simulink model "FullModel"  (R2025b)
settings: Solver=ode15s  StartTime=0.0  StopTime=0.3  FixedStep=1e-6  MaxStep=1e-5  RelTol=1e-5  EnableMultiTasking=on
InitFcn:
  | Rs=0.42;
  | Ls=0.96e-3;
  | C_phi=92.1952e-3;
  | poles=8;
  | Rload=15;
values from neighbouring files (symbols this model uses):
  DutyCycleBoost = 0.7    [run_specification.m]
  Lm = 27.27e-6    (= 2.727e-05)    [run_specification.m]
  Lsec = Lp    (= 0.00012957)    [run_specification.m]
  Rp = 0.3117    [run_specification.m]
  rpm_speed = 500    [run_specification.m]
libraries: spsSeriesRLCBranchLib x15, spsDiodeLib x11, spsVoltageMeasurementLib x7, spsMosfetLib x6, spsControlledVoltageSourceLib x3, spsCurrentMeasurementLib x2, spsPWMGeneratorDCDCLib x2, spsParallelRLCBranchLib x2, spsGroundLib x1, spspowerguiLib x1
settings Model: Creator=jwjansen  LastModifiedBy=20231741
settings SolverCC: AlgebraicLoopSolver=TrustRegion
settings DataIOCC: LimitDataPoints=on  SaveFormat=Array  ReturnWorkspaceOutputs=off
settings OptimizationCC: ExpressionDepthLimit=2147483647.0  LifeSpan=inf
settings DebuggingCC: UnderspecifiedInitializationDetection=Classic  MergeDetectMultiDrivingBlocksExec=none  SolverPrmCheckMsg=warning  FcnCallInpInsideContextMsg=warning  StateNameClashWarn=warning  SFUnexpectedBacktrackingDiag=warning  SFNoUnconditionalDefaultTransitionDiag=warning  SFExecutionAtInitializationDiag=none  ArithmeticOperatorsInVariantConditions=warning
settings HardwareCC: ProdBitPerPointer=32.0  ProdBitPerSizeT=32.0  ProdBitPerPtrDiffT=32.0  ProdLargestAtomicFloat=None  ProdIntDivRoundTo=Undefined  ProdEndianess=Unspecified  ProdWordSize=32.0  ProdHWDeviceType=32-bit Generic
settings ModelReferenceCC: EnableRefExpFcnMdlSchedulingChecks=on  PropagateSignalLabelsOutOfModel=off
settings SFSimCC: SimUseLocalCustomCode=off  SimParseCustomCode=off  CustomCodeUndefinedFunction=UseInterfaceOnly
settings RTWCC: RTWUseLocalCustomCode=off  GPUComputeCapability=3.5
settings CodeAppCC: StateflowObjectComments=on
settings GRTTargetCC: TargetLangStandard=C89/C90 (ANSI)  CombineOutputUpdateFcns=off  GRTInterface=on
settings ConfigComp: CovMetricSettings=dw  CovSaveCumulativeToWorkspaceVar=on  CovSaveSingleToWorkspaceVar=on  CovExternalEMLEnable=off
settings SimscapeCC: SimscapeNormalizeSystem=off

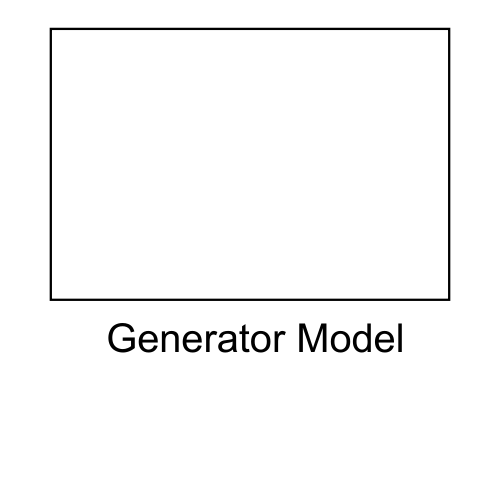
[thumbnail: Simulink's stored preview of the top-level diagram]
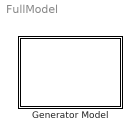
== system FullModel ==
  " Generator Model " : Subsystem

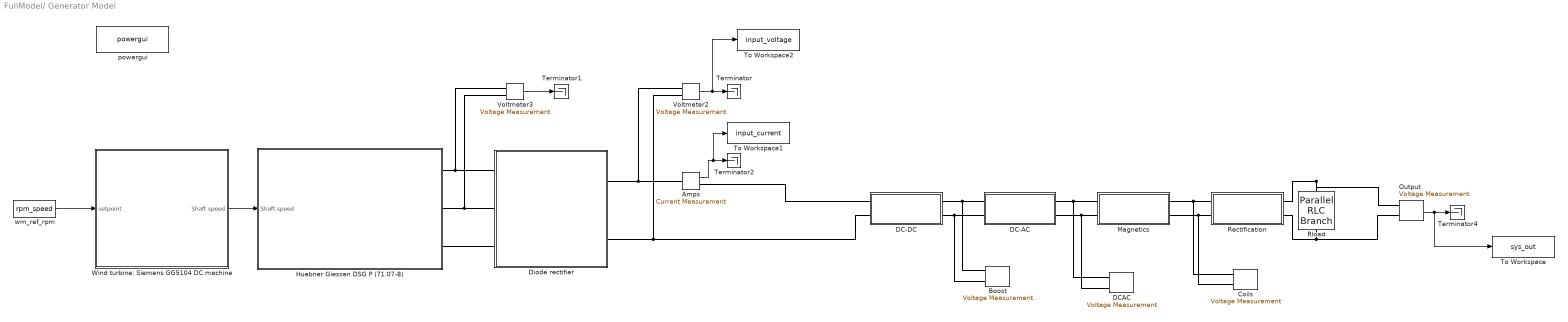
== system FullModel/ Generator Model  ==
  Amps : spsCurrentMeasurementLib/Current Measurement  PhasorSimulation=off  OutputType=Complex  PSBequivalent=0
  Boost : spsVoltageMeasurementLib/Voltage Measurement  PhasorSimulation=off  OutputType=Complex  PSBequivalent=0
  Coils : spsVoltageMeasurementLib/Voltage Measurement  PhasorSimulation=off  OutputType=Complex  PSBequivalent=0
  DC-AC : Subsystem
  DC-DC : Subsystem
  DCAC : spsVoltageMeasurementLib/Voltage Measurement  PhasorSimulation=off  OutputType=Complex  PSBequivalent=0
  Diode rectifier : Subsystem
  "Huebner Giessen DSG P (71.07-8) " : Subsystem
  Magnetics : Subsystem
  Output : spsVoltageMeasurementLib/Voltage Measurement  PhasorSimulation=off  OutputType=Complex  PSBequivalent=0
  Rectification : Subsystem
  Rload : spsParallelRLCBranchLib/Parallel RLC Branch  LConnTagsString=a  RConnTagsString=__new0  BranchType=R  Resistance=9.8  Inductance=0.1e-3  SetiL0=off  InitialCurrent=0  Capacitance=1e-3  Setx0=on  InitialVoltage=14  Measurements=Branch voltage and current
  Terminator{,1..2,4} (4 alike) : Terminator
  To Workspace : ToWorkspace  VariableName=sys_out  SaveFormat=Timeseries  SampleTime=-1
  To Workspace1 : ToWorkspace  VariableName=input_current  SaveFormat=Timeseries  SampleTime=-1
  To Workspace2 : ToWorkspace  VariableName=input_voltage  SaveFormat=Timeseries  SampleTime=-1
  Voltmeter2 : spsVoltageMeasurementLib/Voltage Measurement  PhasorSimulation=off  OutputType=Complex  PSBequivalent=0
  Voltmeter3 : spsVoltageMeasurementLib/Voltage Measurement  PhasorSimulation=off  OutputType=Complex  PSBequivalent=0
  "Wind turbine: Siemens GG5104 DC machine " : Subsystem
  powergui : spspowerguiLib/powergui  Priority=1  SimulationMode=Continuous  SampleTime=1e-6  frequency=60  Iterations=50  frequencyindice=0  Pbase=100e6  ErrMax=1e-4  UnitsV=kV  UnitsW=MW  buscounter=0  FunctionMessages=off  echomessages=off  EnableUseOfTLC=off  CurrentSourceSwitches=off  DisableSnubberDevices=off  DisableRonSwitches=off  DisableVfSwitches=off  DisplayEquations=off  AutomaticDiscreteSolvers=off  SolverType=Tustin  Interpol=off  ExternalGateDelay=off  methode=off  Ts=0  x0status=blocks  SPID=off  SwTol=0  HookPort=off  NonlinearTolerance=1e-4  nMaxIteration=100  ContinueOnMaxIteration=off  RestoreLinks=warning  ResistiveCurrentMeasurement=off  Frange=[0:2:500]  Ylog=off  Xlog=on  ShowGrid=off  save=off  variable=ZData  structure=0  ZoomFFT=off  StartTime=0.0  cycles=1  DisplayStyle=1  fundamental=60  FreqAxis=off  MaxFrequency=1000  frequencyindicesteady=1  RmsSteady=1  display=off
  wm_ref_rpm : Constant  Value=rpm_speed
  wires:
  wm_ref_rpm/1 -> "Wind turbine: Siemens GG5104 DC machine "/1(setpoint)
  "Wind turbine: Siemens GG5104 DC machine "/1(Shaft speed) -> "Huebner Giessen DSG P (71.07-8) "/1(Shaft speed)
  Voltmeter2/1 -> To Workspace2/1, Terminator/1
  Voltmeter3/1 -> Terminator1/1
  Amps/1 -> To Workspace1/1, Terminator2/1
  Output/1 -> To Workspace/1, Terminator4/1
  connections:
  "Huebner Giessen DSG P (71.07-8) "/RConn1 -- Voltmeter3/LConn1 -- Diode rectifier/LConn1
  Diode rectifier/LConn2 -- Voltmeter3/LConn2 -- "Huebner Giessen DSG P (71.07-8) "/RConn2
  Diode rectifier/LConn3 -- "Huebner Giessen DSG P (71.07-8) "/RConn3
  Voltmeter2/LConn1 -- Amps/LConn1 -- Diode rectifier/RConn1
  Voltmeter2/LConn2 -- DC-DC/LConn2 -- Diode rectifier/RConn2
  DC-DC/LConn1 -- Amps/RConn1
  DC-AC/LConn2 -- Boost/LConn2 -- DC-DC/RConn2
  DC-AC/LConn1 -- Boost/LConn1 -- DC-DC/RConn1
  Magnetics/LConn1 -- DCAC/LConn1 -- DC-AC/RConn1
  Magnetics/LConn2 -- DCAC/LConn2 -- DC-AC/RConn2
  Rectification/LConn1 -- Magnetics/RConn1 -- Coils/LConn1
  Rectification/LConn2 -- Magnetics/RConn2 -- Coils/LConn2
  Rload/LConn1 -- Rectification/RConn1 -- Output/LConn1
  Rload/RConn1 -- Rectification/RConn2 -- Output/LConn2

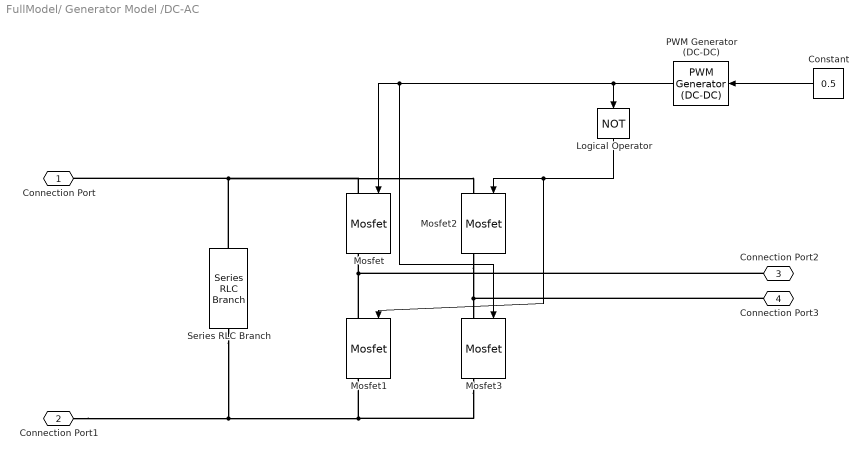
== system FullModel/ Generator Model /DC-AC ==
  Constant : Constant  Value=0.5
  Logical Operator : Logic  Operator=NOT  AllPortsSameDT=off  OutDataTypeStr=boolean
  Mosfet{,1..3} (4 alike) : spsMosfetLib/Mosfet  Ron=90e-3  Lon=0  Rd=0.01  Vfd=0.9  IC=0  Rs=1e5  Cs=inf  Measurements=on
  PWM Generator (DC-DC) : spsPWMGeneratorDCDCLib/PWM Generator (DC-DC)  Fsw=Finv  Ts=0
  Series RLC Branch : spsSeriesRLCBranchLib/Series RLC Branch  LConnTagsString=__new0  RConnTagsString=__new0  BranchType=C  Resistance=1  Inductance=1e-3  SetiL0=off  InitialCurrent=0  Capacitance=470e-6  Setx0=off  InitialVoltage=0  Measurements=None
  Connection Port : PMIOPort  Side=Left
  Connection Port1 : PMIOPort  Port=2  Side=Left
  Connection Port2 : PMIOPort  Port=3  Side=Right
  Connection Port3 : PMIOPort  Port=4  Side=Right
  wires:
  PWM Generator (DC-DC)/1 -> Logical Operator/1, Mosfet3/1, Mosfet/1
  Logical Operator/1 -> Mosfet1/1, Mosfet2/1
  Constant/1 -> PWM Generator (DC-DC)/1
  connections:
  Connection Port1/RConn1 -- Series RLC Branch/RConn1 -- Mosfet3/RConn1 -- Mosfet1/RConn1
  Mosfet2/LConn1 -- Mosfet/LConn1 -- Series RLC Branch/LConn1 -- Connection Port/RConn1
  Connection Port2/RConn1 -- Mosfet/RConn1 -- Mosfet1/LConn1
  Connection Port3/RConn1 -- Mosfet2/RConn1 -- Mosfet3/LConn1

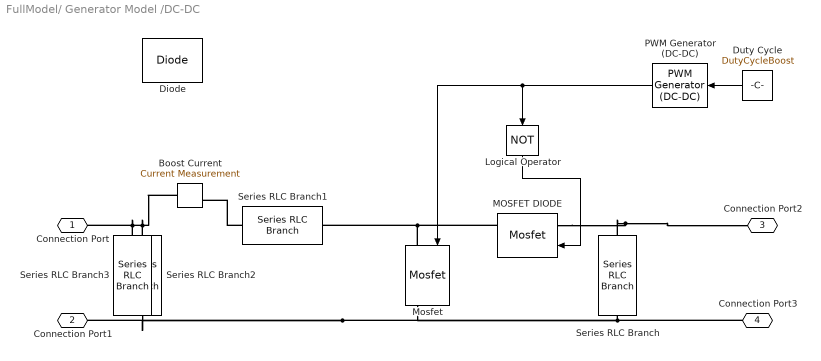
== system FullModel/ Generator Model /DC-DC ==
  Boost Current : spsCurrentMeasurementLib/Current Measurement  PhasorSimulation=off  OutputType=Complex  PSBequivalent=0
  Diode : spsDiodeLib/Diode  Ron=0.001  Lon=0  Vf=0.8  IC=0  UseSnubber=0  Rs=500  Cs=250e-9  Measurements=on
  Duty Cycle : Constant  Value=DutyCycleBoost
  Logical Operator : Logic  Operator=NOT  AllPortsSameDT=off  OutDataTypeStr=boolean
  MOSFET DIODE : spsMosfetLib/Mosfet  Ron=0.0175  Lon=0  Rd=0.01  Vfd=0.9  IC=0  Rs=1e5  Cs=inf  Measurements=on
  Mosfet : spsMosfetLib/Mosfet  Ron=0.0175  Lon=0  Rd=0.01  Vfd=0.9  IC=0  Rs=1e5  Cs=inf  Measurements=on
  PWM Generator (DC-DC) : spsPWMGeneratorDCDCLib/PWM Generator (DC-DC)  Fsw=Fboost  Ts=0
  Series RLC Branch : spsSeriesRLCBranchLib/Series RLC Branch  LConnTagsString=__new0  RConnTagsString=__new0  BranchType=C  Resistance=1  Inductance=0  SetiL0=off  InitialCurrent=0  Capacitance=2200e-6  Setx0=on  InitialVoltage=10  Measurements=None
  Series RLC Branch1 : spsSeriesRLCBranchLib/Series RLC Branch  LConnTagsString=__new0  RConnTagsString=__new0  BranchType=L  Resistance=1  Inductance=100e-6  SetiL0=off  InitialCurrent=0  Capacitance=0  Setx0=off  InitialVoltage=0  Measurements=None
  Series RLC Branch2 : spsSeriesRLCBranchLib/Series RLC Branch  LConnTagsString=__new0  RConnTagsString=__new0  BranchType=C  Resistance=1  Inductance=0  SetiL0=off  InitialCurrent=0  Capacitance=470e-6  Setx0=on  InitialVoltage=10  Measurements=None
  Series RLC Branch3 : spsSeriesRLCBranchLib/Series RLC Branch  LConnTagsString=__new0  RConnTagsString=__new0  BranchType=C  Resistance=1  Inductance=0  SetiL0=off  InitialCurrent=0  Capacitance=470e-6  Setx0=on  InitialVoltage=10  Measurements=None
  Connection Port : PMIOPort  Side=Left
  Connection Port1 : PMIOPort  Port=2  Side=Left
  Connection Port2 : PMIOPort  Port=3  Side=Right
  Connection Port3 : PMIOPort  Port=4  Side=Right
  wires:
  Duty Cycle/1 -> PWM Generator (DC-DC)/1
  PWM Generator (DC-DC)/1 -> Logical Operator/1, Mosfet/1
  Logical Operator/1 -> MOSFET DIODE/1
  connections:
  Series RLC Branch1/RConn1 -- Boost Current/RConn1
  Series RLC Branch/LConn1 -- MOSFET DIODE/LConn1 -- Connection Port2/RConn1
  Mosfet/RConn1 -- Series RLC Branch2/RConn1 -- Connection Port1/RConn1 -- Connection Port3/RConn1 -- Series RLC Branch/RConn1
  Mosfet/LConn1 -- Series RLC Branch1/LConn1 -- MOSFET DIODE/RConn1
  Boost Current/LConn1 -- Series RLC Branch2/LConn1 -- Series RLC Branch3/LConn1 -- Connection Port/RConn1

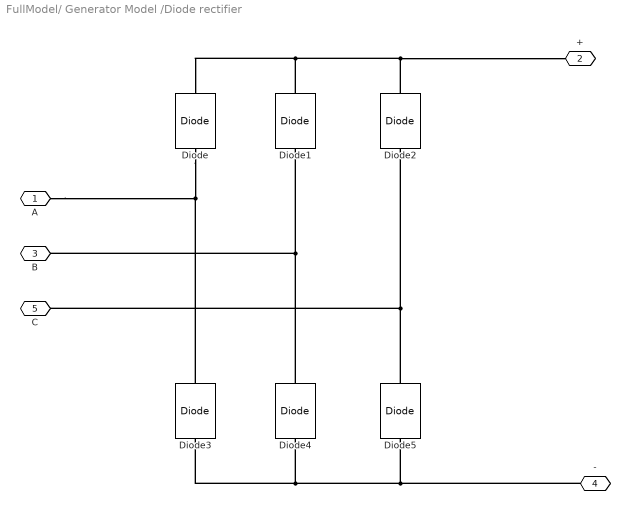
== system FullModel/ Generator Model /Diode rectifier ==
  Diode{,1..5} (6 alike) : spsDiodeLib/Diode  Ron=0.01  Lon=0  Vf=0.85  IC=0  UseSnubber=off  Rs=500  Cs=250e-9  Measurements=off
  A : PMIOPort  Side=Left
  + : PMIOPort  Port=2  Side=Right
  B : PMIOPort  Port=3  Side=Left
  - : PMIOPort  Port=4  Side=Right
  C : PMIOPort  Port=5  Side=Left
  connections:
  Diode2/LConn1 -- C/RConn1 -- Diode5/RConn1
  +/RConn1 -- Diode2/RConn1 -- Diode1/RConn1 -- Diode/RConn1
  Diode3/LConn1 -- -/RConn1 -- Diode5/LConn1 -- Diode4/LConn1
  Diode3/RConn1 -- A/RConn1 -- Diode/LConn1
  Diode1/LConn1 -- B/RConn1 -- Diode4/RConn1

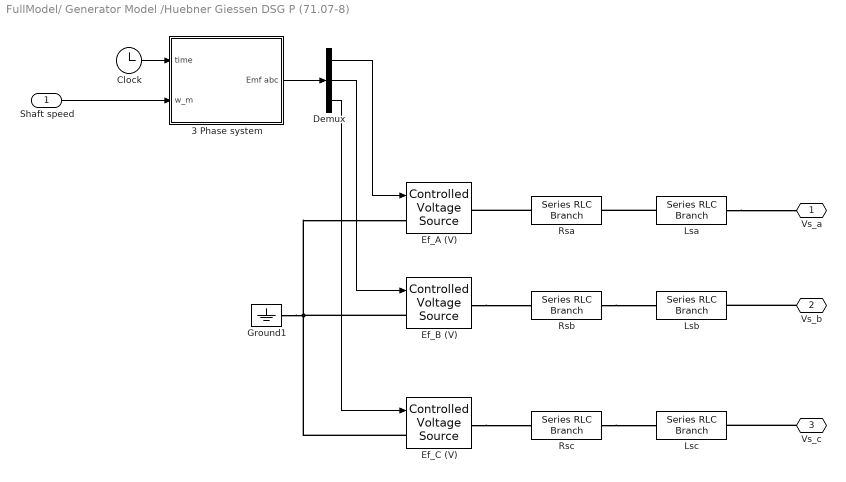
== system FullModel/ Generator Model /Huebner Giessen DSG P (71.07-8)  ==
  Shaft speed : Inport
  "3 Phase system " : Subsystem
  Clock : Clock
  Demux : Demux  Outputs=3
  Ef_A (V) : spsControlledVoltageSourceLib/Controlled Voltage Source  Initialize=on  Source_Type=AC  Amplitude=0  Phase=0  Frequency=0  Measurements=None
  Ef_B (V) : spsControlledVoltageSourceLib/Controlled Voltage Source  Initialize=on  Source_Type=AC  Amplitude=0  Phase=0  Frequency=0  Measurements=None
  Ef_C (V) : spsControlledVoltageSourceLib/Controlled Voltage Source  Initialize=on  Source_Type=AC  Amplitude=0  Phase=0  Frequency=0  Measurements=None
  Ground1 : spsGroundLib/Ground  LConnTagsString=a
  Lsa : spsSeriesRLCBranchLib/Series RLC Branch  LConnTagsString=__new0  RConnTagsString=__new0  BranchType=L  Resistance=Rs  Inductance=Ls  SetiL0=off  InitialCurrent=0  Capacitance=1e-6  Setx0=off  InitialVoltage=0  Measurements=Branch current
  Lsb : spsSeriesRLCBranchLib/Series RLC Branch  LConnTagsString=__new0  RConnTagsString=__new0  BranchType=L  Resistance=Rs  Inductance=Ls  SetiL0=off  InitialCurrent=0  Capacitance=1e-6  Setx0=off  InitialVoltage=0  Measurements=Branch current
  Lsc : spsSeriesRLCBranchLib/Series RLC Branch  LConnTagsString=__new0  RConnTagsString=__new0  BranchType=L  Resistance=Rs  Inductance=Ls  SetiL0=on  InitialCurrent=0  Capacitance=1e-6  Setx0=off  InitialVoltage=0  Measurements=Branch current
  Rsa : spsSeriesRLCBranchLib/Series RLC Branch  LConnTagsString=__new0  RConnTagsString=__new0  BranchType=R  Resistance=Rs  Inductance=Ls  SetiL0=off  InitialCurrent=0  Capacitance=1e-6  Setx0=off  InitialVoltage=0  Measurements=Branch current
  Rsb : spsSeriesRLCBranchLib/Series RLC Branch  LConnTagsString=__new0  RConnTagsString=__new0  BranchType=R  Resistance=Rs  Inductance=Ls  SetiL0=off  InitialCurrent=0  Capacitance=1e-6  Setx0=off  InitialVoltage=0  Measurements=Branch current
  Rsc : spsSeriesRLCBranchLib/Series RLC Branch  LConnTagsString=__new0  RConnTagsString=__new0  BranchType=R  Resistance=Rs  Inductance=Ls  SetiL0=on  InitialCurrent=0  Capacitance=1e-6  Setx0=off  InitialVoltage=0  Measurements=Branch current
  Vs_a : PMIOPort  Side=Right
  Vs_b : PMIOPort  Port=2  Side=Right
  Vs_c : PMIOPort  Port=3  Side=Right
  wires:
  Demux/1 -> Ef_A (V)/1
  Demux/3 -> Ef_C (V)/1
  Demux/2 -> Ef_B (V)/1
  Shaft speed/1 -> "3 Phase system "/2(w_m)
  Clock/1 -> "3 Phase system "/1(time)
  "3 Phase system "/1("Emf abc ") -> Demux/1
  connections:
  Ef_B (V)/RConn1 -- Rsb/LConn1
  Lsa/RConn1 -- Vs_a/RConn1
  Vs_b/RConn1 -- Lsb/RConn1
  Ef_B (V)/LConn1 -- Ground1/LConn1 -- Ef_C (V)/LConn1 -- Ef_A (V)/LConn1
  Vs_c/RConn1 -- Lsc/RConn1
  Lsa/LConn1 -- Rsa/RConn1
  Ef_C (V)/RConn1 -- Rsc/LConn1
  Rsa/LConn1 -- Ef_A (V)/RConn1
  Rsb/RConn1 -- Lsb/LConn1
  Rsc/RConn1 -- Lsc/LConn1

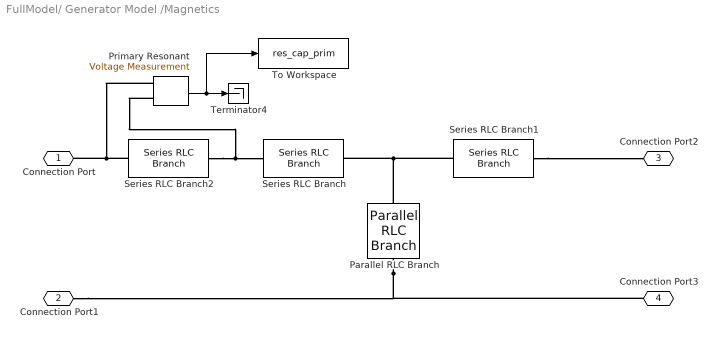
== system FullModel/ Generator Model /Magnetics ==
  Parallel RLC Branch : spsParallelRLCBranchLib/Parallel RLC Branch  LConnTagsString=a  RConnTagsString=__new0  BranchType=L  Resistance=1  Inductance=Lm  SetiL0=off  InitialCurrent=0  Capacitance=1e-6  Setx0=off  InitialVoltage=0  Measurements=None
  Primary Resonant : spsVoltageMeasurementLib/Voltage Measurement  PhasorSimulation=off  OutputType=Complex  PSBequivalent=0
  Series RLC Branch : spsSeriesRLCBranchLib/Series RLC Branch  LConnTagsString=__new0  RConnTagsString=__new0  BranchType=RL  Resistance=Rp  Inductance=Lp - Lm  SetiL0=off  InitialCurrent=0  Capacitance=0  Setx0=off  InitialVoltage=0  Measurements=None
  Series RLC Branch1 : spsSeriesRLCBranchLib/Series RLC Branch  LConnTagsString=__new0  RConnTagsString=__new0  BranchType=RLC  Resistance=Rs  Inductance=Lsec-Lm  SetiL0=off  InitialCurrent=0  Capacitance=47e-9/2  Setx0=off  InitialVoltage=0  Measurements=None
  Series RLC Branch2 : spsSeriesRLCBranchLib/Series RLC Branch  LConnTagsString=__new0  RConnTagsString=__new0  BranchType=C  Resistance=Rp  Inductance=Lp - Lm  SetiL0=off  InitialCurrent=0  Capacitance=47e-9/2  Setx0=off  InitialVoltage=0  Measurements=None
  Terminator4 : Terminator
  To Workspace : ToWorkspace  VariableName=res_cap_prim  SaveFormat=Timeseries  SampleTime=-1
  Connection Port : PMIOPort  Side=Left
  Connection Port1 : PMIOPort  Port=2  Side=Left
  Connection Port2 : PMIOPort  Port=3  Side=Right
  Connection Port3 : PMIOPort  Port=4  Side=Right
  wires:
  Primary Resonant/1 -> To Workspace/1, Terminator4/1
  connections:
  Parallel RLC Branch/RConn1 -- Connection Port3/RConn1 -- Connection Port1/RConn1
  Parallel RLC Branch/LConn1 -- Series RLC Branch1/RConn1 -- Series RLC Branch/RConn1
  Series RLC Branch1/LConn1 -- Connection Port2/RConn1
  Series RLC Branch2/LConn1 -- Primary Resonant/LConn1 -- Connection Port/RConn1
  Series RLC Branch2/RConn1 -- Primary Resonant/LConn2 -- Series RLC Branch/LConn1

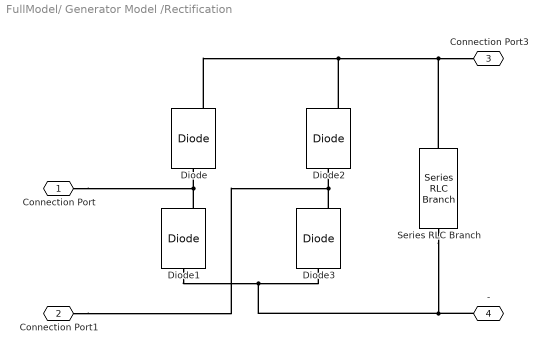
== system FullModel/ Generator Model /Rectification ==
  Diode{,1..3} (4 alike) : spsDiodeLib/Diode  Ron=0.001  Lon=0  Vf=0.8  IC=0  UseSnubber=0  Rs=500  Cs=250e-9  Measurements=on
  Series RLC Branch : spsSeriesRLCBranchLib/Series RLC Branch  LConnTagsString=__new0  RConnTagsString=__new0  BranchType=C  Resistance=1  Inductance=1e-3  SetiL0=off  InitialCurrent=0  Capacitance=10e-6  Setx0=off  InitialVoltage=0  Measurements=None
  Connection Port : PMIOPort  Side=Left
  Connection Port1 : PMIOPort  Port=2  Side=Left
  Connection Port3 : PMIOPort  Port=3  Side=Right
  - : PMIOPort  Port=4  Side=Right
  connections:
  Diode/RConn1 -- Diode2/RConn1 -- Series RLC Branch/LConn1 -- Connection Port3/RConn1
  Connection Port/RConn1 -- Diode1/RConn1 -- Diode/LConn1
  Diode1/LConn1 -- -/RConn1 -- Series RLC Branch/RConn1 -- Diode3/LConn1
  Diode3/RConn1 -- Connection Port1/RConn1 -- Diode2/LConn1

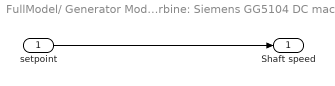
== system FullModel/ Generator Model /Wind turbine: Siemens GG5104 DC machine  ==
  setpoint : Inport
  Shaft speed : Outport
  wires:
  setpoint/1 -> Shaft speed/1

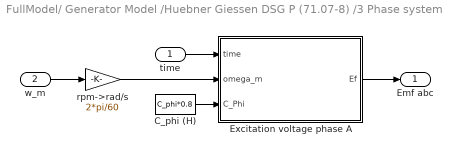
== system FullModel/ Generator Model /Huebner Giessen DSG P (71.07-8) /3 Phase system  ==
  time : Inport
  w_m : Inport  Port=2
  C_phi (H) : Constant  Value=C_phi*0.8  VectorParams1D=off
  Excitation voltage phase A : Subsystem
  rpm->rad/s : Gain  Gain=2*pi/60
  "Emf abc " : Outport
  wires:
  w_m/1 -> rpm->rad/s/1
  C_phi (H)/1 -> Excitation voltage phase A/3(C_Phi)
  time/1 -> Excitation voltage phase A/1(time)
  rpm->rad/s/1 -> Excitation voltage phase A/2(omega_m)
  Excitation voltage phase A/1(Ef) -> "Emf abc "/1

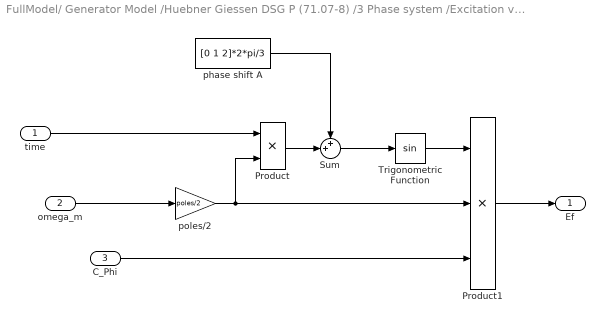
== system FullModel/ Generator Model /Huebner Giessen DSG P (71.07-8) /3 Phase system /Excitation voltage phase A ==
  time : Inport
  omega_m : Inport  Port=2
  C_Phi : Inport  Port=3
  Product : Product  RndMeth=Zero
  Product1 : Product  Inputs=3  RndMeth=Zero
  Sum : Sum  Inputs=++|
  Trigonometric Function : Trigonometry
  phase shift A : Constant  Value=[0 1 2]*2*pi/3
  poles/2 : Gain  Gain=poles/2
  Ef : Outport
  wires:
  poles/2/1 -> Product/2, Product1/2
  Trigonometric Function/1 -> Product1/1
  phase shift A/1 -> Sum/1
  Product/1 -> Sum/2
  Product1/1 -> Ef/1
  C_Phi/1 -> Product1/3
  Sum/1 -> Trigonometric Function/1
  time/1 -> Product/1
  omega_m/1 -> poles/2/1
